simulink model "phi2_narmamaglev_expanded_breach"  (R2017a)
settings: Solver=ode45  StartTime=0.0  StopTime=tspan(end)  RelTol=1e-3  AbsTol=1e-6
model workspace: external: MAT-File /home/nikhil/breach_master/Examples/June2018/narmamaglev_expanded_params.mat (data not in the file)
undefined symbols (not defined in the file or in its folder): B1, B2, B3, B4, IW1_1, IW3_2, IW5_3, LW2_1, LW4_3, LW5_4, LW6_2, LW6_5, max_i, maxp, maxt, min_i, minp, mint, Ni, Nj, Normalize, Ts, u_ts
settings Model: ExtModeTrigMode=oneshot  ExtModeArmWhenConnect=off  TunableVars=prueba  TunableVarsStorageClass=Auto  Creator=The MathWorks Inc.  LastModifiedBy=nikhil
settings DataIOCC: ExternalInput=[t__, u__]  LoadExternalInput=on  SaveFormat=StructureWithTime  ReturnWorkspaceOutputs=on
settings OptimizationCC: BooleanDataType=off  DefaultParameterBehavior=Inlined  ExpressionDepthLimit=2147483647  InitFltsAndDblsToZero=on  LifeSpan=inf
settings DebuggingCC: SaveWithParameterizedLinksMsg=none  UnderspecifiedInitializationDetection=Classic  MergeDetectMultiDrivingBlocksExec=none  SignalResolutionControl=TryResolveAllWithWarning  MultiTaskDSMMsg=warning  MultiTaskCondExecSysMsg=none  FcnCallInpInsideContextMsg=warning  StateNameClashWarn=warning  SFUnexpectedBacktrackingDiag=warning  SFNoUnconditionalDefaultTransitionDiag=warning  SFExecutionAtInitializationDiag=none
settings HardwareCC: ProdBitPerPointer=32  ProdBitPerSizeT=32  ProdBitPerPtrDiffT=32  ProdLargestAtomicFloat=None  ProdIntDivRoundTo=Undefined  ProdEndianess=Unspecified  ProdWordSize=32  ProdHWDeviceType=32-bit Generic  TargetUnknown=on
settings ModelReferenceCC: PropagateSignalLabelsOutOfModel=off
settings RTWCC: TemplateMakefile=grt_vc.tmf
settings GRTTargetCC: TargetFcnLib=ansi_tfl_tmw.mat  TargetLangStandard=C89/C90 (ANSI)  GeneratePreprocessorConditionals=Disable all  CombineOutputUpdateFcns=off  GRTInterface=on
settings ConfigComp: CovMetricSettings=dw  CovHtmlReporting=on  CovSaveCumulativeToWorkspaceVar=on  CovSaveSingleToWorkspaceVar=on  CovExternalEMLEnable=off

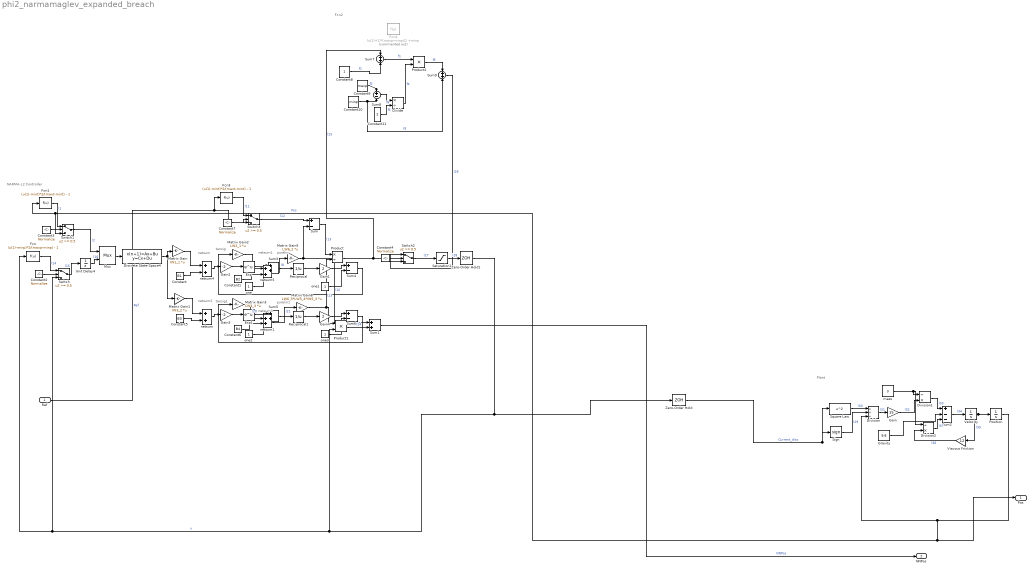
== system phi2_narmamaglev_expanded_breach ==
  note: Fcn2
  note: tansig1
  note: tansig
  note: purelin1
  note: purelin
  note: netsum3
  note: netsum2
  note: netsum1
  note: netsum
  note: Plant
  note: NARMA-L2 Controller
  Ref : Inport
  Constant : Constant  Value=B1
  Constant1 : Constant  Value=B2
  Constant10 : Constant  Value=minp
  Constant11 : Constant  Value=2
  Constant{2..4,7} (4 alike) : Constant  Value=Normalize
  Constant5 : Constant  Value=B3
  Constant6 : Constant  Value=B4
  Constant8 : Constant
  Constant9 : Constant  Value=maxp
  Discrete State-Space4 : DiscreteStateSpace  A=blkdiag([zeros(1,Nj-1);eye(Nj-2,Nj-2) zeros(Nj-2,1)],[zeros(1,Ni-1);eye(Ni-2,Ni-2) zeros(Ni-2,1)])  B=blkdiag(eye(Nj-1,1),eye(Ni-1,1))  C=blkdiag([zeros(1,Nj-1);eye(Nj-1,Nj-1)],[zeros(eye(double(Ni>1)),Ni-1);eye(Ni-2,Ni-1)])  D=blkdiag([1;zeros(Nj-1,1)],[eye(double(Ni>1));zeros(Ni-2,1)])  SampleTime=Ts
  Divide : Product  Inputs=*/
  Division : Product  Inputs=**/  SaturateOnIntegerOverflow=on  InputSameDT=on  OutDataTypeStr=Inherit: Same as first input
  Division1 : Product  Inputs=/*  SaturateOnIntegerOverflow=on  InputSameDT=on  OutDataTypeStr=Inherit: Same as first input
  Division2 : Product  Inputs=/*  SaturateOnIntegerOverflow=on  InputSameDT=on  OutDataTypeStr=Inherit: Same as first input
  Exp : Math  SaturateOnIntegerOverflow=on
  Exp1 : Math  SaturateOnIntegerOverflow=on
  Fcn : Fcn  Expr=(u(1)-minp)*2/(maxp-minp) - 1
  Fcn1 : Fcn  Expr=(u(1)-mint)*2/(maxt-mint) - 1
  Fcn3 : Fcn  Expr=(u(1)-mint)*2/(maxt-mint) - 1
  Fcn4 : Fcn  Commented=on  Expr=(u(1)+1)*(maxp-minp)/2 +minp
  Gain : Gain  Gain=15  SaturateOnIntegerOverflow=on  OutDataTypeStr=Inherit: Same as input  ParamDataTypeStr=Inherit: Same as input
  Gain1 : Gain  Gain=2  SaturateOnIntegerOverflow=on  OutDataTypeStr=Inherit: Same as input  ParamDataTypeStr=Inherit: Same as input
  Gain2 : Gain  Gain=-2  SaturateOnIntegerOverflow=on  OutDataTypeStr=Inherit: Same as input  ParamDataTypeStr=Inherit: Same as input
  Gain3 : Gain  Gain=-2  SaturateOnIntegerOverflow=on  OutDataTypeStr=Inherit: Same as input  ParamDataTypeStr=Inherit: Same as input
  Gain4 : Gain  Gain=2  SaturateOnIntegerOverflow=on  OutDataTypeStr=Inherit: Same as input  ParamDataTypeStr=Inherit: Same as input
  Gravity : Constant  Value=9.8
  Matrix Gain : Gain  Gain=IW1_1  Multiplication=Matrix(K*u)  SaturateOnIntegerOverflow=on  OutDataTypeStr=Inherit: Same as input  ParamDataTypeStr=Inherit: Same as input
  Matrix Gain1 : Gain  Gain=IW3_2  Multiplication=Matrix(K*u)  SaturateOnIntegerOverflow=on  OutDataTypeStr=Inherit: Same as input  ParamDataTypeStr=Inherit: Same as input
  Matrix Gain2 : Gain  Gain=LW2_1  Multiplication=Matrix(K*u)  SaturateOnIntegerOverflow=on  OutDataTypeStr=Inherit: Same as input  ParamDataTypeStr=Inherit: Same as input
  Matrix Gain3 : Gain  Gain=LW4_3  Multiplication=Matrix(K*u)  SaturateOnIntegerOverflow=on  OutDataTypeStr=Inherit: Same as input  ParamDataTypeStr=Inherit: Same as input
  Matrix Gain5 : Gain  Gain=LW6_2  Multiplication=Matrix(K*u)  SaturateOnIntegerOverflow=on  OutDataTypeStr=Inherit: Same as input  ParamDataTypeStr=Inherit: Same as input
  Matrix Gain8 : Gain  Gain=LW6_5*LW5_4*IW5_3  Multiplication=Matrix(K*u)  SaturateOnIntegerOverflow=on  OutDataTypeStr=Inherit: Same as input  ParamDataTypeStr=Inherit: Same as input
  Mux : Mux  Inputs=2
      settings: DisplayOption=signals
  Position : Integrator  InitialCondition=0.5  ZeroCross=off
  Product : Product  Inputs=*/  SaturateOnIntegerOverflow=on  InputSameDT=on  OutDataTypeStr=Inherit: Same as first input
  Product1 : Product  SaturateOnIntegerOverflow=on  InputSameDT=on  OutDataTypeStr=Inherit: Same as first input
  Product2 : Product
  Reciprocal : Math  Operator=reciprocal  SaturateOnIntegerOverflow=on
  Reciprocal1 : Math  Operator=reciprocal  SaturateOnIntegerOverflow=on
  Saturation1 : Saturate  UpperLimit=max_i  LowerLimit=min_i  ZeroCross=off
  Sign : Signum  ZeroCross=off
  Square Law : Fcn  Expr=u^2
  Sum : Sum  Inputs=+-  SaturateOnIntegerOverflow=on  InputSameDT=on  OutDataTypeStr=Inherit: Same as first input
  Sum1 : Sum  SaturateOnIntegerOverflow=on  InputSameDT=on  OutDataTypeStr=Inherit: Same as first input
  Sum2 : Sum  Inputs=|+--  SaturateOnIntegerOverflow=on  InputSameDT=on  OutDataTypeStr=Inherit: Same as first input
  Sum3 : Sum  SaturateOnIntegerOverflow=on  InputSameDT=on  OutDataTypeStr=Inherit: Same as first input
  Sum4 : Sum  Inputs=+-  SaturateOnIntegerOverflow=on  InputSameDT=on  OutDataTypeStr=Inherit: Same as first input
  Sum5 : Sum  SaturateOnIntegerOverflow=on  InputSameDT=on  OutDataTypeStr=Inherit: Same as first input
  Sum6 : Sum  Inputs=+-  SaturateOnIntegerOverflow=on  InputSameDT=on  OutDataTypeStr=Inherit: Same as first input
  Sum7 : Sum
  Sum8 : Sum  Inputs=+-
  Sum9 : Sum
  Switch{,1..3} (4 alike) : Switch  Threshold=0.5  ZeroCross=off  SaturateOnIntegerOverflow=on  InputSameDT=on
  Unit Delay4 : UnitDelay  SampleTime=Ts
  Velocity : Integrator  ZeroCross=off
  Viscous Friction : Gain  Gain=12  SaturateOnIntegerOverflow=on  OutDataTypeStr=Inherit: Same as input  ParamDataTypeStr=Inherit: Same as input
  Zero-Order Hold : ZeroOrderHold  SampleTime=u_ts
  Zero-Order Hold1 : ZeroOrderHold  SampleTime=Ts
  mass : Constant  Value=3
  netsum{,1,4..5} (4 alike) : Sum  Inputs=2  SaturateOnIntegerOverflow=on  InputSameDT=on  OutDataTypeStr=Inherit: Same as first input
  one{,1..3} (4 alike) : Constant
  Pos : Outport
  NNPos : Outport  Port=2
  wires:
  Ref/1 -> Switch3/3, Fcn3/1  "Ref"
  Position/1 -> Fcn1/1, Switch1/3, Pos/1, Division/3  "Pos"
  Zero-Order Hold/1 -> Square Law/1, Sign/1  "Current_disc"
  Sum1/1 -> NNPos/1  "NNPos"
  Product1/1 -> Sum1/2  "l24"
  Switch2/1 -> Saturation1/1  "l27"
  Constant4/1 -> Switch2/2
  Product/1 -> Sum7/1, Switch2/3  "l25"
  Saturation1/1 -> Zero-Order Hold1/1  "l28"
  Switch/1 -> Unit Delay4/1  "l15"
  Unit Delay4/1 -> Mux/2  "l16"
  Constant2/1 -> Switch/2
  Fcn/1 -> Switch/1  "l14"
  Zero-Order Hold1/1 -> Zero-Order Hold/1, Fcn/1, Switch/3, Product1/2  "u"
  Discrete State-Space4/1 -> Matrix Gain/1, Matrix Gain1/1
  Mux/1 -> Discrete State-Space4/1
  Switch1/1 -> Mux/1  "l2"
  Switch3/1 -> Sum/1  "l12"
  Fcn3/1 -> Switch3/1  "l11"
  Constant7/1 -> Switch3/2
  Matrix Gain8/1 -> Product1/1, Product/2  "l23"
  Sum/1 -> Product/1  "l13"
  Matrix Gain5/1 -> Sum/2, Sum1/1  "l10"
  Sum6/1 -> Matrix Gain3/1
  Matrix Gain3/1 -> netsum1/1  "l20"
  netsum1/1 -> Matrix Gain8/1  "l21"
  Sum4/1 -> Matrix Gain2/1
  netsum5/1 -> Matrix Gain5/1  "l8"
  Fcn1/1 -> Switch1/1  "l1"
  Constant3/1 -> Switch1/2
  Sign/1 -> Division/2  "l29"
  Division2/1 -> Sum2/3  "l37"
  Viscous Friction/1 -> Division2/2  "l36"
  mass/1 -> Division1/1, Division2/1
  Division1/1 -> Sum2/1  "l33"
  Gain/1 -> Division1/2  "l32"
  Sum2/1 -> Velocity/1  "l34"
  Velocity/1 -> Position/1, Viscous Friction/1  "l35"
  Gravity/1 -> Sum2/2
  Division/1 -> Gain/1  "l31"
  Square Law/1 -> Division/1  "l30"
  Constant/1 -> netsum4/2
  Matrix Gain/1 -> netsum4/1
  Constant1/1 -> netsum5/2
  Matrix Gain2/1 -> netsum5/1
  Constant5/1 -> netsum/2
  Matrix Gain1/1 -> netsum/1
  Constant6/1 -> netsum1/2
  one1/1 -> Sum4/2
  Gain1/1 -> Sum4/1
  Reciprocal/1 -> Gain1/1
  Sum3/1 -> Reciprocal/1
  one/1 -> Sum3/2
  Exp/1 -> Sum3/1
  Gain2/1 -> Exp/1
  netsum4/1 -> Gain2/1
  one3/1 -> Sum6/2
  Gain4/1 -> Sum6/1
  Reciprocal1/1 -> Gain4/1
  Sum5/1 -> Reciprocal1/1
  one2/1 -> Sum5/2
  Exp1/1 -> Sum5/1
  Gain3/1 -> Exp1/1
  netsum/1 -> Gain3/1
  Product2/1 -> Sum9/1  "f5"
  Divide/1 -> Product2/2  "f4"
  Constant11/1 -> Divide/2  "f4"
  Sum8/1 -> Divide/1  "f6"
  Constant10/1 -> Sum9/2, Sum8/2  "f3"
  Constant9/1 -> Sum8/1  "f2"
  Sum7/1 -> Product2/1  "f1"
  Constant8/1 -> Sum7/2  "f1"
  Sum9/1 -> Switch2/1  "l26"
